simulink model "observer_estimator"  (R2020a)
settings: Solver=VariableStepAuto  StartTime=0.0  StopTime=200  RelTol=1e-13  AbsTol=1e-8
InitFcn:
  | d1=-2;d2=3;
  | Q=[0 1 0;0 0 1;0 -1 0];
  | C=[1 0 0];
  | K=place(Q',C',[-2 -3 -4]);
  | L=K';
settings Model: Creator=Haris  LastModifiedBy=Haris

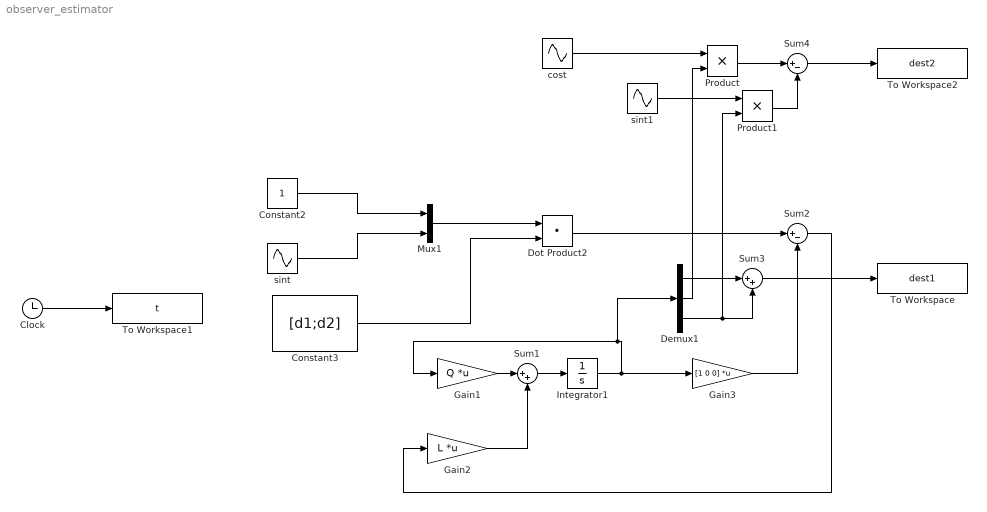
== system observer_estimator ==
  Clock : Clock
  Constant2 : Constant
  Constant3 : Constant  Value=[d1;d2]
  Demux1 : Demux  Outputs=3
  Dot Product2 : DotProduct  InputSameDT=on  OutDataTypeStr=Inherit: Inherit via internal rule
  Gain1 : Gain  Gain=Q  Multiplication=Matrix(K*u)
  Gain2 : Gain  Gain=L  Multiplication=Matrix(K*u)
  Gain3 : Gain  Gain=[1 0 0]  Multiplication=Matrix(K*u)
  Integrator1 : Integrator  InitialCondition=[0;0;0]
  Mux1 : Mux  Inputs=2
  Product : Product
  Product1 : Product
  Sum1 : Sum  Inputs=|++
  Sum2 : Sum  Inputs=|+-
  Sum3 : Sum  Inputs=|++
  Sum4 : Sum  Inputs=|+-
  To Workspace : ToWorkspace  VariableName=dest1  SampleTime=-1
  To Workspace1 : ToWorkspace  VariableName=t  SampleTime=-1
  To Workspace2 : ToWorkspace  VariableName=dest2  SampleTime=-1
  cost : Sin  Phase=pi/2  SampleTime=0
  sint : Sin  SampleTime=0
  sint1 : Sin  SampleTime=0
  wires:
  Clock/1 -> To Workspace1/1
  Gain1/1 -> Sum1/1
  Sum1/1 -> Integrator1/1
  Gain2/1 -> Sum1/2
  Gain3/1 -> Sum2/2
  Constant3/1 -> Dot Product2/2
  Mux1/1 -> Dot Product2/1
  Dot Product2/1 -> Sum2/1
  Constant2/1 -> Mux1/1
  sint/1 -> Mux1/2
  Sum2/1 -> Gain2/1
  Integrator1/1 -> Gain3/1, Demux1/1, Gain1/1
  Demux1/1 -> Sum3/1
  Demux1/3 -> Product1/2, Sum3/2
  Sum3/1 -> To Workspace/1
  cost/1 -> Product/1
  Demux1/2 -> Product/2
  Product/1 -> Sum4/1
  Product1/1 -> Sum4/2
  sint1/1 -> Product1/1
  Sum4/1 -> To Workspace2/1
